simulink model "check_serial_2msg_processor"  (R2021a)
settings: Solver=FixedStepDiscrete  StartTime=0.0  StopTime=inf  FixedStep=time_step  RelTol=1e-3
model workspace (MAT data in the model file):
  time_step = 0.01
undefined symbols (not defined in the file or in its folder): Serial_Port, Standard_Devices
libraries: sldrtlib x4
settings Model: OrderedModelArguments=off  Creator=Rahul Subramanian  LastModifiedBy=Rahul Subramanian
settings SolverCC: AlgebraicLoopSolver=TrustRegion
settings DebuggingCC: SFMachineParentedDataDiag=warning
settings RTWCC: Description=Simulink Desktop Real-Time  SystemTargetFile=sldrt.tlc  TemplateMakefile=sldrt.tmf  RTWCompilerOptimization=on
settings CodeAppCC: MaxIdLength=95
settings SimulinkDesktopRealTimeCC: TargetPreCompLibLocation=C:\Program Files\MATLAB\R2021a\toolbox\sldrt\lib\win64

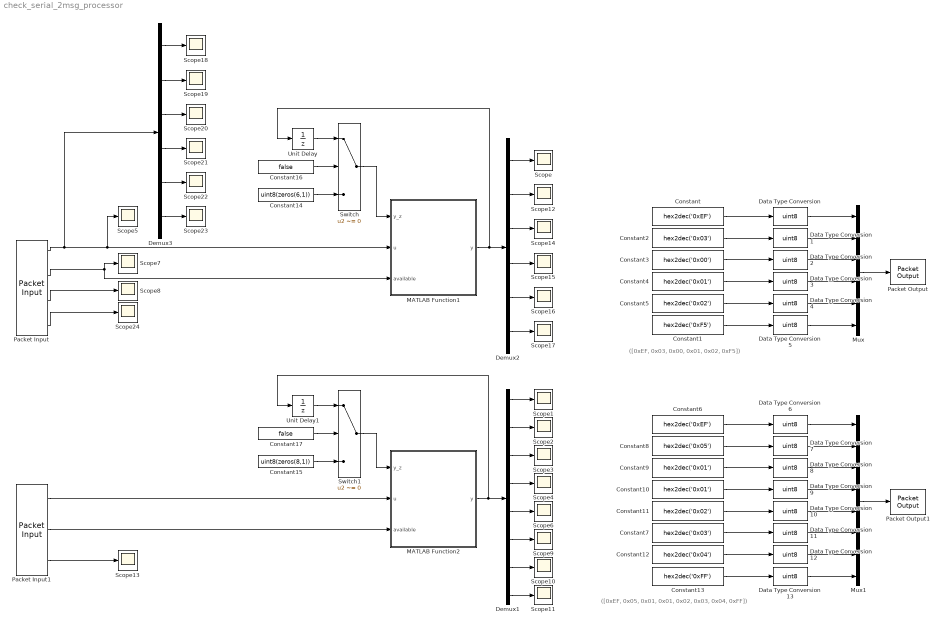
== system check_serial_2msg_processor ==
  note: ([0xEF, 0x05, 0x01, 0x01, 0x02, 0x03, 0x04, 0xFF])
  note: ([0xEF, 0x03, 0x00, 0x01, 0x02, 0xF5])
  Constant : Constant  Value=hex2dec('0xEF')
  Constant1 : Constant  Value=hex2dec('0xF5')
  Constant10 : Constant  Value=hex2dec('0x01')
  Constant11 : Constant  Value=hex2dec('0x02')
  Constant12 : Constant  Value=hex2dec('0x04')
  Constant13 : Constant  Value=hex2dec('0xFF')
  Constant14 : Constant  Value=uint8(zeros(6,1))
  Constant15 : Constant  Value=uint8(zeros(8,1))
  Constant16 : Constant  Value=false
  Constant17 : Constant  Value=false
  Constant2 : Constant  Value=hex2dec('0x03')
  Constant3 : Constant  Value=hex2dec('0x00')
  Constant4 : Constant  Value=hex2dec('0x01')
  Constant5 : Constant  Value=hex2dec('0x02')
  Constant6 : Constant  Value=hex2dec('0xEF')
  Constant7 : Constant  Value=hex2dec('0x03')
  Constant8 : Constant  Value=hex2dec('0x05')
  Constant9 : Constant  Value=hex2dec('0x01')
  Data Type Conversion{,1..13} (14 alike) : DataTypeConversion  OutDataTypeStr=uint8
  Demux1 : Demux  Outputs=8
  Demux2 : Demux  Outputs=6
  Demux3 : Demux  Outputs=6
  MATLAB Function1 : MATLAB Function  TreatAsAtomicUnit=on
  MATLAB Function2 : MATLAB Function  TreatAsAtomicUnit=on
  Mux : Mux  Inputs=6
  Mux1 : Mux  Inputs=8
  Packet Input : sldrtlib/Packet Input  SampleTime=time_step  MaxMissedTicks=inf  ShowMissedTicks=on  YieldWhenWaiting=off  DrvName=Standard_Devices/Serial_Port  DrvAddress=5  DrvOptions=[115200 8 0 0 0 0 0 0]  PacketSize=6  DataTypes='6*uint8'  ShowReady=on  ShowError=on  PacketID=1  ByteOrder=1  ShowTimestamp=off
      settings: AttributesFormatString=Serial Port [5]
  Packet Input1 : sldrtlib/Packet Input  SampleTime=time_step  MaxMissedTicks=inf  ShowMissedTicks=on  YieldWhenWaiting=off  DrvName=Standard_Devices/Serial_Port  DrvAddress=5  DrvOptions=[115200 8 0 0 0 0 0 0]  PacketSize=8  DataTypes='8*uint8'  ShowReady=on  ShowError=off  PacketID=1  ByteOrder=1  ShowTimestamp=off
      settings: AttributesFormatString=Serial Port [5]
  Packet Output : sldrtlib/Packet Output  SampleTime=time_step  MaxMissedTicks=inf  ShowMissedTicks=off  YieldWhenWaiting=off  DrvName=Standard_Devices/Serial_Port  DrvAddress=5  DrvOptions=[115200 8 0 0 0 0 0 0]  PacketSize=6  DataTypes='6*uint8'  ShowReady=off  ShowError=off  PacketID=1  ByteOrder=1  InitialValue=[]  FinalValue=[]
      settings: AttributesFormatString=Serial Port [5]
  Packet Output1 : sldrtlib/Packet Output  SampleTime=time_step  MaxMissedTicks=inf  ShowMissedTicks=off  YieldWhenWaiting=off  DrvName=Standard_Devices/Serial_Port  DrvAddress=5  DrvOptions=[115200 8 0 0 0 0 0 0]  PacketSize=8  DataTypes='8*uint8'  ShowReady=off  ShowError=off  PacketID=1  ByteOrder=1  InitialValue=[]  FinalValue=[]
      settings: AttributesFormatString=Serial Port [5]
  Scope{,1..24} (25 alike) : Scope
  Switch : Switch  Criteria=u2 ~= 0
  Switch1 : Switch  Criteria=u2 ~= 0
  Unit Delay : UnitDelay  SampleTime=-1  HasFrameUpgradeWarning=on
  Unit Delay1 : UnitDelay  SampleTime=-1  HasFrameUpgradeWarning=on
  wires:
  Constant/1 -> Data Type Conversion/1
  Constant2/1 -> Data Type Conversion1/1
  Constant3/1 -> Data Type Conversion2/1
  Constant4/1 -> Data Type Conversion3/1
  Constant5/1 -> Data Type Conversion4/1
  Data Type Conversion/1 -> Mux/1
  Data Type Conversion1/1 -> Mux/2
  Data Type Conversion2/1 -> Mux/3
  Data Type Conversion3/1 -> Mux/4
  Data Type Conversion4/1 -> Mux/5
  Packet Input/3 -> Scope8/1
  Mux/1 -> Packet Output/1
  Constant1/1 -> Data Type Conversion5/1
  Data Type Conversion5/1 -> Mux/6
  Data Type Conversion11/1 -> Mux1/6
  Constant7/1 -> Data Type Conversion11/1
  Mux1/1 -> Packet Output1/1
  Data Type Conversion10/1 -> Mux1/5
  Data Type Conversion9/1 -> Mux1/4
  Data Type Conversion8/1 -> Mux1/3
  Data Type Conversion7/1 -> Mux1/2
  Data Type Conversion6/1 -> Mux1/1
  Constant11/1 -> Data Type Conversion10/1
  Constant10/1 -> Data Type Conversion9/1
  Constant9/1 -> Data Type Conversion8/1
  Constant8/1 -> Data Type Conversion7/1
  Constant6/1 -> Data Type Conversion6/1
  Data Type Conversion12/1 -> Mux1/7
  Data Type Conversion13/1 -> Mux1/8
  Constant12/1 -> Data Type Conversion12/1
  Constant13/1 -> Data Type Conversion13/1
  Demux2/1 -> Scope/1
  MATLAB Function1/1(y) -> Unit Delay/1, Demux2/1
  Demux2/2 -> Scope12/1
  Demux2/3 -> Scope14/1
  Demux2/4 -> Scope15/1
  Demux2/5 -> Scope16/1
  Demux2/6 -> Scope17/1
  Switch/1 -> MATLAB Function1/1(y_z)
  Demux1/6 -> Scope9/1
  Demux1/5 -> Scope6/1
  Demux1/4 -> Scope4/1
  Demux1/3 -> Scope3/1
  Demux1/2 -> Scope2/1
  MATLAB Function2/1(y) -> Unit Delay1/1, Demux1/1
  Demux1/1 -> Scope1/1
  Packet Input/2 -> MATLAB Function1/3(available), Scope7/1
  Demux1/8 -> Scope11/1
  Demux1/7 -> Scope10/1
  Packet Input1/1 -> MATLAB Function2/2(u)
  Packet Input1/2 -> MATLAB Function2/3(available)
  Unit Delay/1 -> Switch/1
  Constant16/1 -> Switch/2
  Constant14/1 -> Switch/3
  Constant15/1 -> Switch1/3
  Constant17/1 -> Switch1/2
  Unit Delay1/1 -> Switch1/1
  Switch1/1 -> MATLAB Function2/1(y_z)
  Packet Input1/3 -> Scope13/1
  Demux3/6 -> Scope23/1
  Demux3/5 -> Scope22/1
  Demux3/4 -> Scope21/1
  Demux3/3 -> Scope20/1
  Demux3/2 -> Scope19/1
  Packet Input/1 -> Demux3/1, MATLAB Function1/2(u), Scope5/1
  Demux3/1 -> Scope18/1
  Packet Input/4 -> Scope24/1

== matlab function check_serial_2msg_processor/MATLAB Function1 ==
  data: y_z input size=6; u input uint8; y output uint8 size=6; available input
function y  = fcn(y_z, u, available)

y = y_z;
data_packet_size = uint8(0);

if available
    if u(1) == hex2dec('0xEF')
        if u(3) == 0
            for j = 1:6
                y(j) = u(j);
            end
    %             data_packet_size = u(2) - 1;
    %             data_id = u(3);
    %             data(1) = u(4);
    %             data(2) = u(5);
    %             crc(3) = u(6);
        end
    end
end

== matlab function check_serial_2msg_processor/MATLAB Function2 ==
  data: y_z input size=8; u input uint8; y output uint8 size=8; available input
function y  = fcn(y_z, u, available)

y = y_z;
data_packet_size = uint8(0);

if available
    if u(1) == hex2dec('0xEF')
        if u(3) == 1
            for j = 1:8
                y(j) = u(j);
            end
    %             data_packet_size = u(2) - 1;
    %             data_id = u(3);
    %             data(1) = u(4);
    %             data(2) = u(5);
    %             crc(3) = u(6);
        end
    end
end
